simulink model "robot_dinamica"  (R2021a)
settings: Solver=ode45  StartTime=0.0  StopTime=2  MaxStep=1e-3  RelTol=1e-3
settings Model: Creator=Pablo Carmona  LastModifiedBy=Pablo Carmona

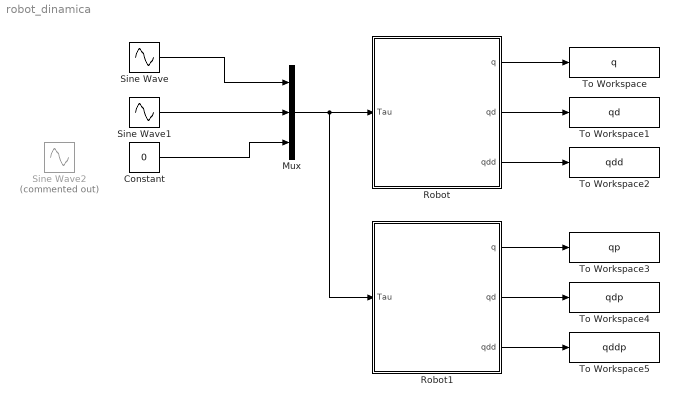
== system robot_dinamica ==
  Constant : Constant  Value=0
  Mux : Mux  Inputs=3
  Robot : Subsystem
      mask Display: image('captura_esquema_3GDL_cleanup.png'); % Use "Edit Image" on toolstrip to change.
  Robot1 : Subsystem
      mask Display: image('esquema3gdl_limpio.jpg'); % Use "Edit Image" on toolstrip to change.
  Sine Wave : Sin  Amplitude=0.5  SampleTime=0
  Sine Wave1 : Sin  Amplitude=0.5  SampleTime=0
  Sine Wave2 : Sin  Commented=on  Frequency=10  SampleTime=0
  To Workspace : ToWorkspace  VariableName=q  SaveFormat=Structure With Time  SampleTime=-1
  To Workspace1 : ToWorkspace  VariableName=qd  SaveFormat=Structure With Time  SampleTime=-1
  To Workspace2 : ToWorkspace  VariableName=qdd  SaveFormat=Structure With Time  SampleTime=-1
  To Workspace3 : ToWorkspace  VariableName=qp  SaveFormat=Structure With Time  SampleTime=-1
  To Workspace4 : ToWorkspace  VariableName=qdp  SaveFormat=Structure With Time  SampleTime=-1
  To Workspace5 : ToWorkspace  VariableName=qddp  SaveFormat=Structure With Time  SampleTime=-1
  wires:
  Mux/1 -> Robot1/1(Tau), Robot/1(Tau)
  Sine Wave/1 -> Mux/1
  Constant/1 -> Mux/3
  Sine Wave1/1 -> Mux/2
  Robot/1(q) -> To Workspace/1
  Robot/2(qd) -> To Workspace1/1
  Robot/3(qdd) -> To Workspace2/1
  Robot1/3(qdd) -> To Workspace5/1
  Robot1/2(qd) -> To Workspace4/1
  Robot1/1(q) -> To Workspace3/1

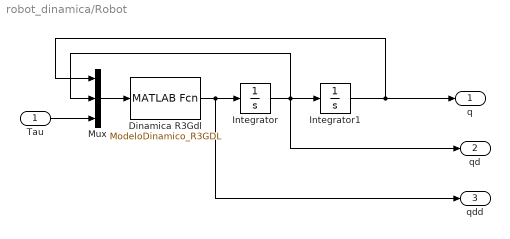
== system robot_dinamica/Robot ==
  Tau : Inport
  Dinamica R3Gdl : MATLABFcn  MATLABFcn=ModeloDinamico_R3GDL  OutputDimensions=3
  Integrator : Integrator  InitialCondition=[0;0;0];
  Integrator1 : Integrator  InitialCondition=[0,0,0]
  Mux : Mux  Inputs=3
  q : Outport
  qd : Outport  Port=2
  qdd : Outport  Port=3
  wires:
  Mux/1 -> Dinamica R3Gdl/1
  Dinamica R3Gdl/1 -> Integrator/1, qdd/1
  Integrator/1 -> Integrator1/1, qd/1, Mux/2
  Integrator1/1 -> q/1, Mux/1
  Tau/1 -> Mux/3

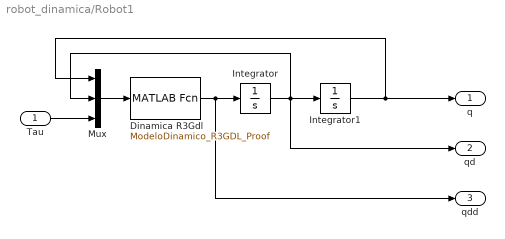
== system robot_dinamica/Robot1 ==
  Tau : Inport
  Dinamica R3Gdl : MATLABFcn  MATLABFcn=ModeloDinamico_R3GDL_Proof  OutputDimensions=3
  Integrator : Integrator  InitialCondition=[0;0;0];
  Integrator1 : Integrator  InitialCondition=[0,0,0]
  Mux : Mux  Inputs=3
  q : Outport
  qd : Outport  Port=2
  qdd : Outport  Port=3
  wires:
  Mux/1 -> Dinamica R3Gdl/1
  Dinamica R3Gdl/1 -> Integrator/1, qdd/1
  Integrator/1 -> Integrator1/1, qd/1, Mux/2
  Integrator1/1 -> q/1, Mux/1
  Tau/1 -> Mux/3
